simulink model "fat"  (R2016b)
settings: Solver=VariableStepAuto  StartTime=0.0  StopTime=15.0  RelTol=1e-3
settings Model: Creator=Roozbeh  LastModifiedBy=Roozbeh

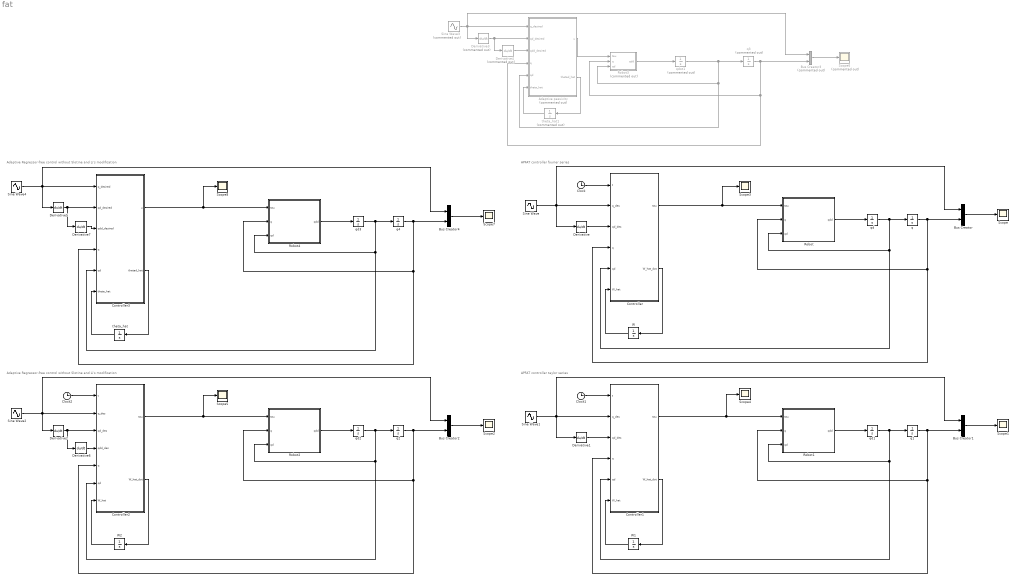
== system fat ==
  note: Adaptive Regressor-free control without Slotine and Li's modification
  note: APFAT controller taylor series
  note: APFAT controller fourier series
  note: Adaptive Regressor-free control without Slotine and Li's modification
  Adaptive passivity : MATLAB Function  Commented=on  TreatAsAtomicUnit=on
  Bus Creator{,1..2,4} (4 alike) : BusCreator  Inputs=2
  Bus Creator3 : BusCreator  Commented=on  Inputs=2
  Clock : Clock
  Clock1 : Clock
  Clock2 : Clock
  Controller : MATLAB Function  TreatAsAtomicUnit=on
  Controller1 : MATLAB Function  TreatAsAtomicUnit=on
  Controller2 : MATLAB Function  TreatAsAtomicUnit=on
  Controller3 : MATLAB Function  TreatAsAtomicUnit=on
  Derivative{,1..2,5..7} (6 alike) : Derivative
  Derivative3 : Derivative  Commented=on
  Derivative4 : Derivative  Commented=on
  Robot : MATLAB Function  TreatAsAtomicUnit=on
  Robot1 : MATLAB Function  TreatAsAtomicUnit=on
  Robot2 : MATLAB Function  TreatAsAtomicUnit=on
  Robot3 : MATLAB Function  Commented=on  TreatAsAtomicUnit=on
  Robot4 : MATLAB Function  TreatAsAtomicUnit=on
  Scope{,1..5,7..8} (8 alike) : Scope
  Scope6 : Scope  Commented=on
  Sine Wave{,1..2,4} (4 alike) : Sin  Amplitude=[1; 0.25; 0.5]  Bias=[0; 0 ; -pi/2]  Frequency=2  SampleTime=0
  Sine Wave3 : Sin  Commented=on  Amplitude=ones(3,1)*0  Bias=ones(3,1)*10  SampleTime=0
  W : Integrator  InitialCondition=zeros(3*9,3)
  W1 : Integrator  InitialCondition=zeros(3*3,3)
  W2 : Integrator  InitialCondition=zeros(3*3,3)
  q{,1..2,4} (4 alike) : Integrator  InitialCondition=[1.2; -1.2; 0.5]
  q3 : Integrator  Commented=on  InitialCondition=[0 0 0]'
  qd{,1..3} (4 alike) : Integrator  InitialCondition=zeros(3,1)
  qdot1 : Integrator  Commented=on  InitialCondition=[0 0 0]'
  theta_hat : Integrator  InitialCondition=zeros(3,1)
  theta_hat1 : Integrator  Commented=on  InitialCondition=|
      | [5.6542
      |     1.1574
      |     2.3321
      |     6.5314
      |     0.6524]'
  wires:
  Controller/1(tau) -> Scope3/1, Robot/1(tau)
  Controller/2(W_hat_dot) -> W/1
  W/1 -> Controller/6(W_hat)
  Robot/1(qdd) -> qd/1
  qd/1 -> Controller/5(qd), Robot/3(qd), q/1
  q/1 -> Bus Creator/2, Controller/4(q), Robot/2(q)
  Sine Wave/1 -> Bus Creator/1, Derivative/1, Controller/2(q_des)
  Derivative/1 -> Controller/3(qd_des)
  Clock/1 -> Controller/1(t)
  Bus Creator/1 -> Scope/1
  Controller1/1(tau) -> Scope4/1, Robot1/1(tau)
  Controller1/2(W_hat_dot) -> W1/1
  W1/1 -> Controller1/6(W_hat)
  Robot1/1(qdd) -> qd1/1
  qd1/1 -> q1/1, Robot1/3(qd), Controller1/5(qd)
  q1/1 -> Robot1/2(q), Controller1/4(q), Bus Creator1/2
  Sine Wave1/1 -> Controller1/2(q_des), Derivative1/1, Bus Creator1/1
  Derivative1/1 -> Controller1/3(qd_des)
  Clock1/1 -> Controller1/1(t)
  Bus Creator1/1 -> Scope1/1
  Controller2/1(tau) -> Scope5/1, Robot2/1(tau)
  Controller2/2(W_hat_dot) -> W2/1
  W2/1 -> Controller2/7(W_hat)
  Robot2/1(qdd) -> qd2/1
  qd2/1 -> Controller2/6(qd), Robot2/3(qd), q2/1
  q2/1 -> Bus Creator2/2, Controller2/5(q), Robot2/2(q)
  Sine Wave2/1 -> Bus Creator2/1, Derivative2/1, Controller2/2(q_des)
  Derivative2/1 -> Derivative6/1, Controller2/3(qd_des)
  Clock2/1 -> Controller2/1(t)
  Bus Creator2/1 -> Scope2/1
  Robot3/1(qdd) -> qdot1/1
  qdot1/1 -> q3/1, Robot3/3(qd), Adaptive passivity/5(qd)
  q3/1 -> Robot3/2(q), Adaptive passivity/4(q), Bus Creator3/2
  Adaptive passivity/1(u) -> Robot3/1(tau)
  Adaptive passivity/2(thetad_hat) -> theta_hat1/1
  theta_hat1/1 -> Adaptive passivity/6(theta_hat)
  Sine Wave3/1 -> Derivative3/1, Bus Creator3/1, Adaptive passivity/1(q_desired)
  Derivative3/1 -> Adaptive passivity/2(qd_desired), Derivative4/1
  Derivative4/1 -> Adaptive passivity/3(qdd_desired)
  Bus Creator3/1 -> Scope6/1
  Derivative6/1 -> Controller2/4(qdd_des)
  Controller3/1(u) -> Scope8/1, Robot4/1(tau)
  Controller3/2(thetad_hat) -> theta_hat/1
  theta_hat/1 -> Controller3/6(theta_hat)
  Robot4/1(qdd) -> qd3/1
  qd3/1 -> Controller3/5(qd), Robot4/3(qd), q4/1
  q4/1 -> Bus Creator4/2, Controller3/4(q), Robot4/2(q)
  Sine Wave4/1 -> Derivative5/1, Bus Creator4/1, Controller3/1(q_desired)
  Derivative5/1 -> Derivative7/1, Controller3/2(qd_desired)
  Bus Creator4/1 -> Scope7/1
  Derivative7/1 -> Controller3/3(qdd_desired)

== matlab function fat/Controller1 ==
  data: t input; q_des input; qd_des input; q input; qd input; W_hat input; tau output; W_hat_dot output
function [tau, W_hat_dot] = fcn(t, q_des, qd_des, q, qd, W_hat)

gamma = diag([6 35 6]);
r = (qd - qd_des) + gamma * (q - q_des);

zz = [1; t; t^2];

Z = [zz' zz' zz']';

K = diag([30 300 30]);

tau = transpose(W_hat)*Z - K*r;

% update
Q = 300*eye(3*3); % 3Bx3B
sigma = 0.009;

W_hat_dot = -pinv(Q)*(Z*transpose(r) + sigma*W_hat); %3Bx3

== matlab function fat/Robot1 ==
  data: tau input; q input; qd input; qdd output
function qdd = fcn(tau, q, qd)

g = 9.81;

theta1 = q(1);
theta2 = q(2);
theta3 = q(3);
qd1 = qd(1);
qd2 = qd(2);
qd3 = qd(3);

G1 = 0;
G2 = -(9*g*(803*cos(theta2)*cos(theta3) - 803*sin(theta2)*sin(theta3) + 4728*sin(theta2)))/10000;
G3 = -(7227*g*(cos(theta2)*cos(theta3) - sin(theta2)*sin(theta3)))/10000;
D11 = ((1300860*cos(theta3)^2 + 5203440*sin(theta3) - 13513230)*cos(theta2)^2)/10000000 - 65043*(7/9 + (sin(theta3) - 4)*sin(theta2))*cos(theta3)*cos(theta2)/500000 - (65043*cos(theta3)^2)/1000000 + ((1011780*sin(theta3) - 5957280)*sin(theta2))/10000000 - (65043*sin(theta3))/125000 + 14294407/10000000;
D12 = 0;
D13 = 0;
D22 = 1351323/1000000 - (65043*sin(theta3))/125000;
D23 = -(65043*sin(theta3))/250000 + 65043/1000000;
D33 = 65043/1000000;
V1 = -(65043*qd1*(cos(theta3)*((qd2 + qd3)*sin(theta3) - 4*qd2 - 2*qd3)*cos(theta2)^2 + (sin(theta2)*(qd2 + qd3)*cos(theta3)^2 + ((4*qd2 + 2*qd3)*sin(theta3) - (16683*qd2)/1606 - qd3/2)*sin(theta2) + (-(7*qd2)/18 - (7*qd3)/18)*sin(theta3) + (5516*qd2)/2409)*cos(theta2) - (7*cos(theta3)*(sin(theta2) + (9*sin(theta3))/7 - 36/7)*(qd2 + qd3))/18))/250000;
V2 = (65043*qd1^2*cos(theta3)^2*cos(theta2)*sin(theta2))/500000 + ((130086*qd1^2*(sin(theta3) - 4)*cos(theta2)^2 - 50589*qd1^2*sin(theta2) - 65043*qd1^2*sin(theta3) + 260172*qd1^2 - 520344*qd3*(qd2 + qd3/2))*cos(theta3))/1000000 + 65043*((sin(theta3) - 16683/6424)*sin(theta2) - (7*sin(theta3))/72 + 1379/2409)*qd1^2*cos(theta2)/125000;
V3 = 65043*(cos(theta3)*(sin(theta3) - 2)*cos(theta2)^2 + (cos(theta3)^2*sin(theta2) + (2*sin(theta3) - 1/2)*sin(theta2) - (7*sin(theta3))/18)*cos(theta2) - 7*(sin(theta2) + (9*sin(theta3))/7 - 36/7)*cos(theta3)/18)*qd1^2/500000 + (65043*qd2^2*cos(theta3))/250000;

G = [G1; G2; G3];
D = [D11 D12 D13; D12 D22 D23; D13 D23 D33];
V = [V1; V2; V3];
F = [qd1; qd2; qd3]*0.05;

qdd = pinv(D)*(tau - V - G - F);

== matlab function fat/Controller2 ==
  data: t input; q_des input; qd_des input; qdd_des input; q input; qd input; W_hat input; tau output; W_hat_dot output
function [tau, W_hat_dot] = fcn(t, q_des, qd_des, qdd_des, q, qd, W_hat)

e = q - q_des;
ed = qd - qd_des;

fn = 3;

zz = [1; cos(fn*t)*sin(fn*t); cos(2*fn*t)*sin(2*fn*t)];

Z = [zz; zz; zz]; % nB

Kd = diag([30 300 30]);
Kp = diag([30 300 30]);

tau = transpose(W_hat)*Z + qdd_des - Kp*e - Kd*ed;

% update
%Q = eye(2*3); % 2n x 2n
%A = [zeros(3) eye(3); -Kp, -Kd];
B = [zeros(3); eye(3)];
%P = lyap(A,Q)
P = [0.5172         0         0   -0.5000         0         0; ...
         0    0.5017         0         0   -0.5000         0; ...
         0         0    0.5172         0         0   -0.5000; ...
   -0.5000         0         0    0.5167         0         0; ...
         0   -0.5000         0         0    0.5017         0; ...
         0         0   -0.5000         0         0    0.5167];

gamma = 300*eye(3*3); % nB x nB
sigma = 0.009;
x = [e; ed];

W_hat_dot = -pinv(gamma)*(Z*transpose(x)*P*B + sigma*W_hat);

== matlab function fat/Robot2 ==
  data: tau input; q input; qd input; qdd output
function qdd = fcn(tau, q, qd)

g = 9.81;

theta1 = q(1);
theta2 = q(2);
theta3 = q(3);
qd1 = qd(1);
qd2 = qd(2);
qd3 = qd(3);

G1 = 0;
G2 = -(9*g*(803*cos(theta2)*cos(theta3) - 803*sin(theta2)*sin(theta3) + 4728*sin(theta2)))/10000;
G3 = -(7227*g*(cos(theta2)*cos(theta3) - sin(theta2)*sin(theta3)))/10000;
D11 = ((1300860*cos(theta3)^2 + 5203440*sin(theta3) - 13513230)*cos(theta2)^2)/10000000 - 65043*(7/9 + (sin(theta3) - 4)*sin(theta2))*cos(theta3)*cos(theta2)/500000 - (65043*cos(theta3)^2)/1000000 + ((1011780*sin(theta3) - 5957280)*sin(theta2))/10000000 - (65043*sin(theta3))/125000 + 14294407/10000000;
D12 = 0;
D13 = 0;
D22 = 1351323/1000000 - (65043*sin(theta3))/125000;
D23 = -(65043*sin(theta3))/250000 + 65043/1000000;
D33 = 65043/1000000;
V1 = -(65043*qd1*(cos(theta3)*((qd2 + qd3)*sin(theta3) - 4*qd2 - 2*qd3)*cos(theta2)^2 + (sin(theta2)*(qd2 + qd3)*cos(theta3)^2 + ((4*qd2 + 2*qd3)*sin(theta3) - (16683*qd2)/1606 - qd3/2)*sin(theta2) + (-(7*qd2)/18 - (7*qd3)/18)*sin(theta3) + (5516*qd2)/2409)*cos(theta2) - (7*cos(theta3)*(sin(theta2) + (9*sin(theta3))/7 - 36/7)*(qd2 + qd3))/18))/250000;
V2 = (65043*qd1^2*cos(theta3)^2*cos(theta2)*sin(theta2))/500000 + ((130086*qd1^2*(sin(theta3) - 4)*cos(theta2)^2 - 50589*qd1^2*sin(theta2) - 65043*qd1^2*sin(theta3) + 260172*qd1^2 - 520344*qd3*(qd2 + qd3/2))*cos(theta3))/1000000 + 65043*((sin(theta3) - 16683/6424)*sin(theta2) - (7*sin(theta3))/72 + 1379/2409)*qd1^2*cos(theta2)/125000;
V3 = 65043*(cos(theta3)*(sin(theta3) - 2)*cos(theta2)^2 + (cos(theta3)^2*sin(theta2) + (2*sin(theta3) - 1/2)*sin(theta2) - (7*sin(theta3))/18)*cos(theta2) - 7*(sin(theta2) + (9*sin(theta3))/7 - 36/7)*cos(theta3)/18)*qd1^2/500000 + (65043*qd2^2*cos(theta3))/250000;

G = [G1; G2; G3];
D = [D11 D12 D13; D12 D22 D23; D13 D23 D33];
V = [V1; V2; V3];
F = [qd1; qd2; qd3]*0.05;

qdd = pinv(D)*(tau - V - G - F);

== matlab function fat/Adaptive passivity ==
  data: q_desired input; qd_desired input; qdd_desired input; q input; u output; qd input; theta_hat input; thetad_hat output
function [u, thetad_hat] = fcn( q_desired, qd_desired, qdd_desired, q, qd,theta_hat)

g = 9.81;
q1 = q(1);
q2 = q(2);
q3 = q(3);

qd1 = qd(1);
qd2 = qd(2);
qd3 = qd(3);

e_q = q - q_desired;
e_qd = qd - qd_desired;

gamma = eye(3);
v = qd_desired - gamma*e_q;
vd = qdd_desired - gamma*e_qd;
r = qd - v;

wn = 10;
Kd = eye(3)*wn^2;
Kp = eye(3)*2*wn;
qdd1 = vd(1);
qdd2 = vd(2);
qdd3 = vd(3);

Y = [qdd1 qdd1 + qdd2 2*qdd1*cos(q2) + qdd2*cos(q2) - v(1)*qd2*sin(q2) - qd1*v(2)*sin(q2) - 2*qd2*v(2)*sin(q2) 0 qdd1 + qdd2; ...
    0 qdd1 + qdd2 qdd1*cos(q2) + qd1*v(1)*sin(q2) 0 qdd1 + qdd2; 0 0 0 qdd3 + g 0];

K = 5*eye(3);
u = Y*theta_hat - K*r;

%update
L = eye(5)*0.2;
thetad_hat = -pinv(L)*transpose(Y)*r;

== matlab function fat/Robot ==
  data: tau input; q input; qd input; qdd output
function qdd = fcn(tau, q, qd)

g = 9.81;

theta1 = q(1);
theta2 = q(2);
theta3 = q(3);
qd1 = qd(1);
qd2 = qd(2);
qd3 = qd(3);

G1 = 0;
G2 = -(9*g*(803*cos(theta2)*cos(theta3) - 803*sin(theta2)*sin(theta3) + 4728*sin(theta2)))/10000;
G3 = -(7227*g*(cos(theta2)*cos(theta3) - sin(theta2)*sin(theta3)))/10000;
D11 = ((1300860*cos(theta3)^2 + 5203440*sin(theta3) - 13513230)*cos(theta2)^2)/10000000 - 65043*(7/9 + (sin(theta3) - 4)*sin(theta2))*cos(theta3)*cos(theta2)/500000 - (65043*cos(theta3)^2)/1000000 + ((1011780*sin(theta3) - 5957280)*sin(theta2))/10000000 - (65043*sin(theta3))/125000 + 14294407/10000000;
D12 = 0;
D13 = 0;
D22 = 1351323/1000000 - (65043*sin(theta3))/125000;
D23 = -(65043*sin(theta3))/250000 + 65043/1000000;
D33 = 65043/1000000;
V1 = -(65043*qd1*(cos(theta3)*((qd2 + qd3)*sin(theta3) - 4*qd2 - 2*qd3)*cos(theta2)^2 + (sin(theta2)*(qd2 + qd3)*cos(theta3)^2 + ((4*qd2 + 2*qd3)*sin(theta3) - (16683*qd2)/1606 - qd3/2)*sin(theta2) + (-(7*qd2)/18 - (7*qd3)/18)*sin(theta3) + (5516*qd2)/2409)*cos(theta2) - (7*cos(theta3)*(sin(theta2) + (9*sin(theta3))/7 - 36/7)*(qd2 + qd3))/18))/250000;
V2 = (65043*qd1^2*cos(theta3)^2*cos(theta2)*sin(theta2))/500000 + ((130086*qd1^2*(sin(theta3) - 4)*cos(theta2)^2 - 50589*qd1^2*sin(theta2) - 65043*qd1^2*sin(theta3) + 260172*qd1^2 - 520344*qd3*(qd2 + qd3/2))*cos(theta3))/1000000 + 65043*((sin(theta3) - 16683/6424)*sin(theta2) - (7*sin(theta3))/72 + 1379/2409)*qd1^2*cos(theta2)/125000;
V3 = 65043*(cos(theta3)*(sin(theta3) - 2)*cos(theta2)^2 + (cos(theta3)^2*sin(theta2) + (2*sin(theta3) - 1/2)*sin(theta2) - (7*sin(theta3))/18)*cos(theta2) - 7*(sin(theta2) + (9*sin(theta3))/7 - 36/7)*cos(theta3)/18)*qd1^2/500000 + (65043*qd2^2*cos(theta3))/250000;

G = [G1; G2; G3];
D = [D11 D12 D13; D12 D22 D23; D13 D23 D33];
V = [V1; V2; V3];
F = [qd1; qd2; qd3]*0.05;

qdd = pinv(D)*(tau - V - G - F);

== matlab function fat/Controller ==
  data: t input; q_des input; qd_des input; q input; qd input; W_hat input; tau output; W_hat_dot output
function [tau, W_hat_dot] = fcn(t, q_des, qd_des, q, qd, W_hat)

gamma = diag([6 35 6]);
r = (qd - qd_des) + gamma * (q - q_des);

fn = 10;
zz = [1; cos(fn*t)*sin(fn*t); cos(2*fn*t)*sin(2*fn*t); cos(3*fn*t)*sin(3*fn*t); cos(4*fn*t)*sin(4*fn*t);...
    cos(5*fn*t)*sin(5*fn*t); cos(6*fn*t)*sin(6*fn*t); cos(7*fn*t)*sin(7*fn*t); cos(8*fn*t)*sin(8*fn*t)];

Z = [zz' zz' zz']';

K = diag([30 300 30]);

tau = transpose(W_hat)*Z - K*r;

% update
Q = 300*eye(3*9); % 3Bx3B
sigma = 0.009;

W_hat_dot = -pinv(Q)*(Z*transpose(r) + sigma*W_hat); %3Bx3

== matlab function fat/Robot3 ==
  data: tau input; qdd output; q input; qd input
function qdd = fcn(tau, q, qd)

a1 = 0.6;
a2 = 0.4;

Lc1 = 0.3;
Lc2 = 0.2;

g = 9.81;
m1 = 12;
m2 = 6;
m3 = 6;
I1 = 0.36;
I2 = 0.36;
I3 = 0.36;

q1 = q(1);
q2 = q(2);
q3 = q(3);
qd1 = qd(1);
qd2 = qd(2);
qd3 = qd(3);

d11 = m1*Lc1^2 + m2*(a1^2 + Lc2^2 + 2*a1*Lc2*cos(q2)) + m3*(a1^2 + a2^2 + 2*a1*a2*cos(q2)) + I1 + I2 + I3;
d12 = m2*(Lc2^2 + a1*Lc2*cos(q2)) + m3*(a2^2 + a1*a2*cos(q2)) + I2 + I3;
d22 = m2*Lc2^2 + m3*a2^2 + I2 + I3;
d13 = 0;
d23 = 0;
d33 = m3;

D = [d11 d12 d13; d12 d22 d23; d13 d23 d33];

h = -m2*a1*Lc2*sin(q2) - m3*a1*a2*sin(q2);
C = [h*qd2 h*qd1+h*qd2 0; -h*qd1 0 0; 0 0 0];

G_mat = [0; 0; m3*g];

qdd = pinv(D)*(tau - C*qd - G_mat);

== matlab function fat/Controller3 ==
  data: q_desired input; qd_desired input; qdd_desired input; q input; qd input; theta_hat input; u output; thetad_hat output
function [u, thetad_hat] = fcn( q_desired, qd_desired, qdd_desired, q, qd,theta_hat)

g = 9.81;
q1 = q(1);
q2 = q(2);
q3 = q(3);

qd1 = qd(1);
qd2 = qd(2);
qd3 = qd(3);

e_q = q - q_desired;
e_qd = qd - qd_desired;

gamma = eye(3);
v = qd_desired - gamma*e_q;
vd = qdd_desired - gamma*e_qd;
r = qd - v;

wn = 10;
Kd = eye(3)*wn^2;
Kp = eye(3)*2*wn;
qdd1 = vd(1);
qdd2 = vd(2);
qdd3 = vd(3);

Y = [qdd1 qdd1 + qdd2 2*qdd1*cos(q2) + qdd2*cos(q2) - v(1)*qd2*sin(q2) - qd1*v(2)*sin(q2) - 2*qd2*v(2)*sin(q2) 0 qdd1 + qdd2; ...
    0 qdd1 + qdd2 qdd1*cos(q2) + qd1*v(1)*sin(q2) 0 qdd1 + qdd2; 0 0 0 qdd3 + g 0];

K = 5*eye(3);
u = Y*theta_hat - K*r;

%update
L = eye(5)*0.2;
thetad_hat = -pinv(L)*transpose(Y)*r;

== matlab function fat/Robot4 ==
  data: tau input; q input; qd input; qdd output
function qdd = fcn(tau, q, qd)

g = 9.81;

theta1 = q(1);
theta2 = q(2);
theta3 = q(3);
qd1 = qd(1);
qd2 = qd(2);
qd3 = qd(3);

G1 = 0;
G2 = -(9*g*(803*cos(theta2)*cos(theta3) - 803*sin(theta2)*sin(theta3) + 4728*sin(theta2)))/10000;
G3 = -(7227*g*(cos(theta2)*cos(theta3) - sin(theta2)*sin(theta3)))/10000;
D11 = ((1300860*cos(theta3)^2 + 5203440*sin(theta3) - 13513230)*cos(theta2)^2)/10000000 - 65043*(7/9 + (sin(theta3) - 4)*sin(theta2))*cos(theta3)*cos(theta2)/500000 - (65043*cos(theta3)^2)/1000000 + ((1011780*sin(theta3) - 5957280)*sin(theta2))/10000000 - (65043*sin(theta3))/125000 + 14294407/10000000;
D12 = 0;
D13 = 0;
D22 = 1351323/1000000 - (65043*sin(theta3))/125000;
D23 = -(65043*sin(theta3))/250000 + 65043/1000000;
D33 = 65043/1000000;
V1 = -(65043*qd1*(cos(theta3)*((qd2 + qd3)*sin(theta3) - 4*qd2 - 2*qd3)*cos(theta2)^2 + (sin(theta2)*(qd2 + qd3)*cos(theta3)^2 + ((4*qd2 + 2*qd3)*sin(theta3) - (16683*qd2)/1606 - qd3/2)*sin(theta2) + (-(7*qd2)/18 - (7*qd3)/18)*sin(theta3) + (5516*qd2)/2409)*cos(theta2) - (7*cos(theta3)*(sin(theta2) + (9*sin(theta3))/7 - 36/7)*(qd2 + qd3))/18))/250000;
V2 = (65043*qd1^2*cos(theta3)^2*cos(theta2)*sin(theta2))/500000 + ((130086*qd1^2*(sin(theta3) - 4)*cos(theta2)^2 - 50589*qd1^2*sin(theta2) - 65043*qd1^2*sin(theta3) + 260172*qd1^2 - 520344*qd3*(qd2 + qd3/2))*cos(theta3))/1000000 + 65043*((sin(theta3) - 16683/6424)*sin(theta2) - (7*sin(theta3))/72 + 1379/2409)*qd1^2*cos(theta2)/125000;
V3 = 65043*(cos(theta3)*(sin(theta3) - 2)*cos(theta2)^2 + (cos(theta3)^2*sin(theta2) + (2*sin(theta3) - 1/2)*sin(theta2) - (7*sin(theta3))/18)*cos(theta2) - 7*(sin(theta2) + (9*sin(theta3))/7 - 36/7)*cos(theta3)/18)*qd1^2/500000 + (65043*qd2^2*cos(theta3))/250000;

G = [G1; G2; G3];
D = [D11 D12 D13; D12 D22 D23; D13 D23 D33];
V = [V1; V2; V3];
F = [qd1; qd2; qd3]*0.05;

qdd = pinv(D)*(tau - V - G - F);
